simulink model "Measure_collection_Vf_W"  (R2021b)
settings: Solver=FixedStepAuto  StartTime=0.0  StopTime=200  FixedStep=1e-2  MaxStep=1e-1  RelTol=1e-2
values from neighbouring files (symbols this model uses):
  Ba = 0.02*ones(3,1)    [sensors_model.m]
  Bg = 5*ones(3,1)    [sensors_model.m]
undefined symbols (not defined in the file or in its folder): B, Spline
libraries: robotcorelib x10
settings Model: Creator=vince  LastModifiedBy=pierg

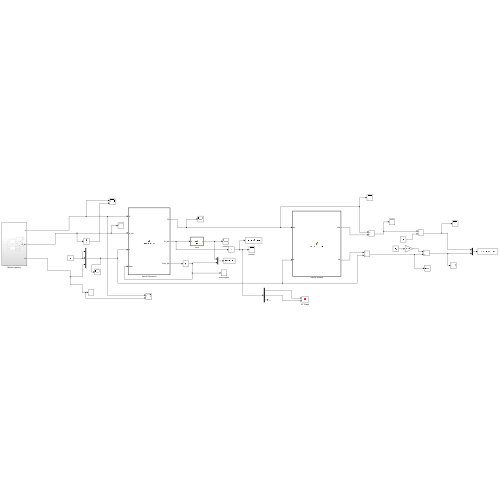
[thumbnail: Simulink's stored preview of the top-level diagram]
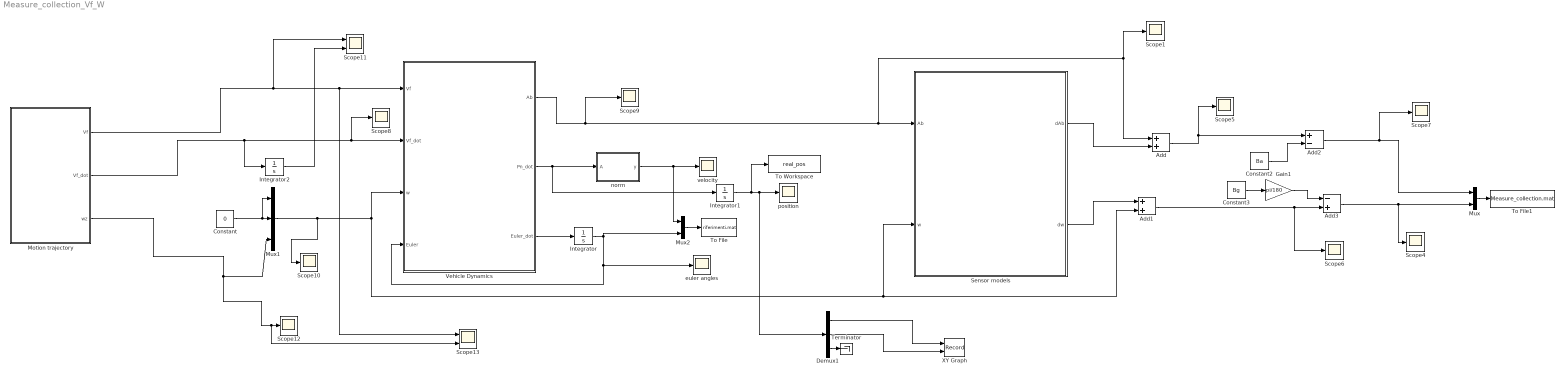
== system Measure_collection_Vf_W ==
  Add : Sum
  Add1 : Sum
  Add2 : Sum  Inputs=+-
  Add3 : Sum  Inputs=-+
  Constant : Constant  Value=0
  Constant2 : Constant  Value=Ba
  Constant3 : Constant  Value=Bg
  Demux1 : Demux  Outputs=3
  Gain1 : Gain  Gain=pi/180
  Integrator : Integrator  InitialCondition=[0 0 pi/2]'
  Integrator1 : Integrator  InitialCondition=[0 0 0]'
  Integrator2 : Integrator
  Motion trajectory : Subsystem
  Mux : Mux  Inputs=2
  Mux1 : Mux  Inputs=3
  Mux2 : Mux  Inputs=2
  Scope{1,4..10,12} (9 alike) : Scope
  Scope11 : Scope  NumInputPorts=2
  Scope13 : Scope  NumInputPorts=2
  Sensor models : MATLAB Function  TreatAsAtomicUnit=on
  Terminator : Terminator
  To File : ToFile  Filename=riferimenti.mat  MatrixName=ground_truth
  To File1 : ToFile  Filename=Measure_collection.mat  MatrixName=measure
  To Workspace : ToWorkspace  VariableName=real_pos  SaveFormat=Structure With Time  SampleTime=-1
  Vehicle Dynamics : MATLAB Function  TreatAsAtomicUnit=on
  XY Graph : Record  FileSettingsInternal="{\"entries\":[{\"content\":{\"excelSettings\":{\"content\":{},\"type\":\"Streamout.ExcelSettings\"}},\"type\":\"Streamout.FileSettingStorage\",\"uuid\":\"d67d7959-5b69-43ab-8784-a510eb5570ce\"}],\"packageUris\":[\"http://schema.mathworks.com/mf0/streamout_blocks/R2020a\"],\"version\":\"1.0\"}"  Layout=[1 1]  SignalsInternal="{\"entries\":[{\"content\":{\"signals\":[{\"content\":{\"blockPath\":[\"Measure_collection_Vf_W/XY Graph\"],\"channel\":[],\"dimensions\":[1,1],\"domain\":\"Measure_collection_Vf_W/XY Graph\",\"lineColor\":\"#a2142f\",\"plots\":[1],\"port\":1,\"sid\":[\"\"],\"signalID\":8310,\"signalName\":\"Demux1:1\"},\"type\":\"RecordBlkView.Signal\",\"uuid\":\"d98b29fb-951e-4e16-8393-070bce4ed298\"},{\"content\":{\"blockPath\":[\"Measure_collection_Vf_W/XY Graph\"],\"channel\":[],\"dimensions\":[1,1],\"domain\":\"Measure_collection_Vf_W/XY Graph\",\"lineColor\":\"#139fff\",\"plots\":[1],\"port\":2,\"sid\":[\"\"],\"signalID\":8314,\"signalName\":\"Demux1:2\"},\"type\":\"RecordBlkView.Signal\",\"uuid\":\"cd6d549f-a1b7-4e28-9178-ba3033d08120\"}]},\"type\":\"RecordBlkView.InputSignals\",\"uuid\":\"81421917-7cfd-46e5-9d72-67f20ea953c8\"}],\"packageUris\":[\"http://schema.mathworks.com/mf0/streamout_blocks/R2020a\"],\"version\":\"1.0\"}"  VisualizationBindings="{\"xyplotplugin\":{\"info\":[{\"series\":[{\"bindingParametersList\":[{\"parameter\":\"X-Axis\",\"signalID\":8310,\"signalName\":\"Demux1:1\"},{\"parameter\":\"Y-Axis\",\"signalID\":8314,\"signalName\":\"Demux1:2\"}],\"seriesID\":35238}],\"subplotID\":1}]}}"  CompatibilityTag=XY
  euler angles : Scope
  norm : MATLAB Function  TreatAsAtomicUnit=on
  position : Scope
  velocity : Scope
  wires:
  Sensor models/1(dAb) -> Add/2
  Mux1/1 -> Scope10/1, Vehicle Dynamics/3(w), Sensor models/2(w), Add1/2
  Sensor models/2(dw) -> Add1/1
  Add/1 -> Add2/1, Scope5/1
  Mux/1 -> To File1/1
  Vehicle Dynamics/3(Euler_dot) -> Integrator/1
  Vehicle Dynamics/2(Pn_dot) -> norm/1(A), Integrator1/1
  Integrator/1 -> Mux2/2, Vehicle Dynamics/4(Euler), euler angles/1
  Add1/1 -> Scope6/1, Add3/2
  Vehicle Dynamics/1(Ab) -> Scope9/1, Scope1/1, Add/1, Sensor models/1(Ab)
  Constant2/1 -> Add2/2
  Add2/1 -> Scope7/1, Mux/1
  Add3/1 -> Scope4/1, Mux/2
  Constant3/1 -> Gain1/1
  Gain1/1 -> Add3/1
  Motion trajectory/2(Vf_dot) -> Integrator2/1, Scope8/1, Vehicle Dynamics/2(Vf_dot)
  Constant/1 -> Mux1/1, Mux1/2
  Motion trajectory/3(wz) -> Mux1/3, Scope13/2, Scope12/1
  Motion trajectory/1(Vf) -> Scope11/1, Vehicle Dynamics/1(Vf), Scope13/1
  Integrator2/1 -> Scope11/2
  norm/1(y) -> Mux2/1, velocity/1
  Demux1/1 -> XY Graph/1
  Integrator1/1 -> To Workspace/1, Demux1/1, position/1
  Demux1/2 -> XY Graph/2
  Demux1/3 -> Terminator/1
  Mux2/1 -> To File/1

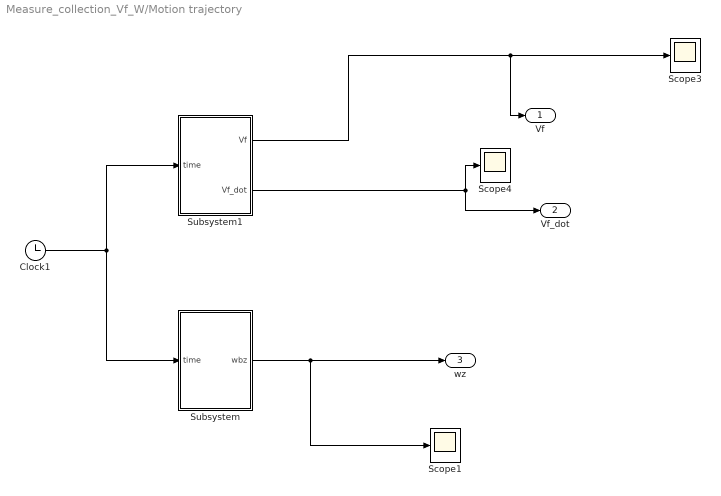
== system Measure_collection_Vf_W/Motion trajectory ==
  Clock1 : Clock
  Scope1 : Scope
  Scope3 : Scope
  Scope4 : Scope
  Subsystem : Subsystem
  Subsystem1 : Subsystem
  Vf : Outport
  Vf_dot : Outport  Port=2
  wz : Outport  Port=3
  wires:
  Clock1/1 -> Subsystem1/1(time), Subsystem/1(time)
  Subsystem1/2(Vf_dot) -> Scope4/1, Vf_dot/1
  Subsystem1/1(Vf) -> Vf/1, Scope3/1
  Subsystem/1(wbz) -> Scope1/1, wz/1

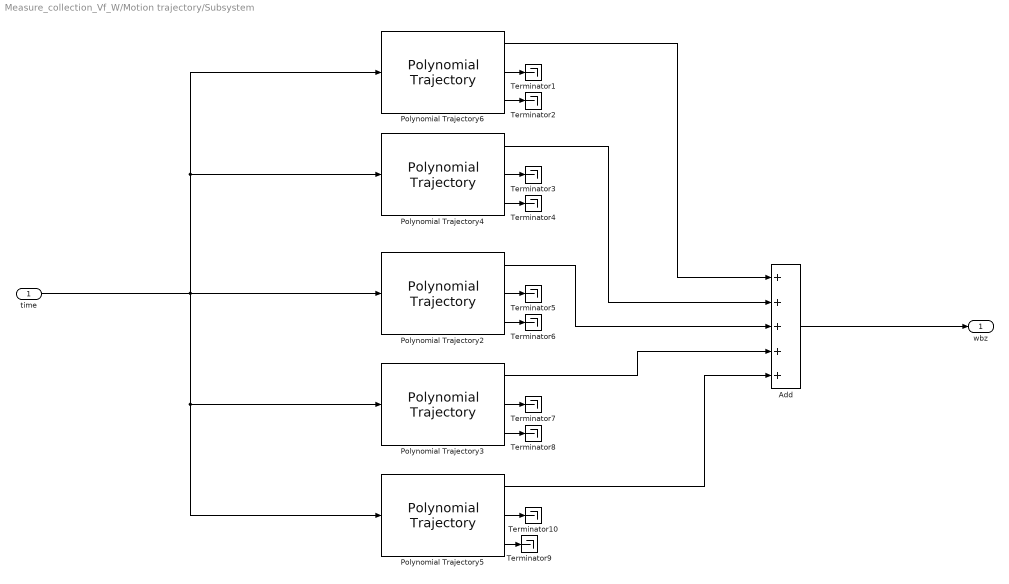
== system Measure_collection_Vf_W/Motion trajectory/Subsystem ==
  time : Inport
  Add : Sum  Inputs=+++++
  Polynomial Trajectory2 : robotcorelib/Polynomial Trajectory  WaypointSource=Internal  Waypoints=wz_des_3  TimePoints=[ 0, 2, 4, , ]  TimeInterval=[75, 115]  Method=B-Spline  ParameterSource=Internal  VelocityBoundaryCondition=zeros( 1, 5 )  AccelerationBoundaryCondition=zeros( 2, 5 )  SimulateUsing=Interpreted execution
  Polynomial Trajectory3 : robotcorelib/Polynomial Trajectory  WaypointSource=Internal  Waypoints=wz_des_4  TimePoints=[ 0, 2, 4, , ]  TimeInterval=[115, 155]  Method=B-Spline  ParameterSource=Internal  VelocityBoundaryCondition=zeros( 1, 5 )  AccelerationBoundaryCondition=zeros( 2, 5 )  SimulateUsing=Interpreted execution
  Polynomial Trajectory4 : robotcorelib/Polynomial Trajectory  WaypointSource=Internal  Waypoints=wz_des_2  TimePoints=[ 0, 2, 4, , ]  TimeInterval=[35, 75]  Method=B-Spline  ParameterSource=Internal  VelocityBoundaryCondition=zeros( 1, 5 )  AccelerationBoundaryCondition=zeros( 2, 5 )  SimulateUsing=Interpreted execution
  Polynomial Trajectory5 : robotcorelib/Polynomial Trajectory  WaypointSource=Internal  Waypoints=wz_des_5  TimePoints=[ 0, 2, 4, , ]  TimeInterval=[155, 200]  Method=B-Spline  ParameterSource=Internal  VelocityBoundaryCondition=zeros( 1, 5 )  AccelerationBoundaryCondition=zeros( 2, 5 )  SimulateUsing=Interpreted execution
  Polynomial Trajectory6 : robotcorelib/Polynomial Trajectory  WaypointSource=Internal  Waypoints=wz_des_1  TimePoints=[ 0, 2, 4, , ]  TimeInterval=[0, 35]  Method=B-Spline  ParameterSource=Internal  VelocityBoundaryCondition=zeros( 1, 5 )  AccelerationBoundaryCondition=zeros( 2, 5 )  SimulateUsing=Interpreted execution
  Terminator{1..10} (10 alike) : Terminator
  wbz : Outport
  wires:
  Polynomial Trajectory2/2 -> Terminator5/1
  Polynomial Trajectory6/1 -> Add/1
  Polynomial Trajectory3/1 -> Add/4
  Polynomial Trajectory4/1 -> Add/2
  Polynomial Trajectory3/3 -> Terminator8/1
  Polynomial Trajectory5/3 -> Terminator9/1
  Polynomial Trajectory6/3 -> Terminator2/1
  Polynomial Trajectory4/2 -> Terminator3/1
  Polynomial Trajectory2/1 -> Add/3
  Polynomial Trajectory5/1 -> Add/5
  Polynomial Trajectory3/2 -> Terminator7/1
  Polynomial Trajectory2/3 -> Terminator6/1
  Polynomial Trajectory5/2 -> Terminator10/1
  Polynomial Trajectory6/2 -> Terminator1/1
  Polynomial Trajectory4/3 -> Terminator4/1
  Add/1 -> wbz/1
  time/1 -> Polynomial Trajectory5/1, Polynomial Trajectory3/1, Polynomial Trajectory2/1, Polynomial Trajectory6/1, Polynomial Trajectory4/1

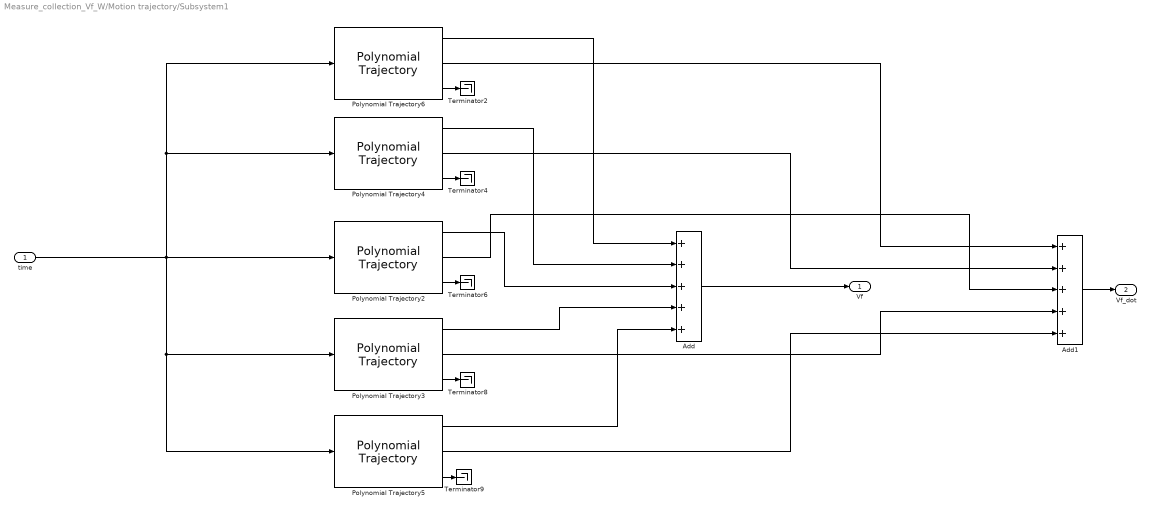
== system Measure_collection_Vf_W/Motion trajectory/Subsystem1 ==
  time : Inport
  Add : Sum  Inputs=+++++
  Add1 : Sum  Inputs=+++++
  Polynomial Trajectory2 : robotcorelib/Polynomial Trajectory  WaypointSource=Internal  Waypoints=Vf_des_3  TimePoints=[ 0, 2, 4, , ]  TimeInterval=[75, 115]  Method=B-Spline  ParameterSource=Internal  VelocityBoundaryCondition=zeros( 1, 5 )  AccelerationBoundaryCondition=zeros( 2, 5 )  SimulateUsing=Interpreted execution
  Polynomial Trajectory3 : robotcorelib/Polynomial Trajectory  WaypointSource=Internal  Waypoints=Vf_des_4  TimePoints=[ 0, 2, 4, , ]  TimeInterval=[115, 155]  Method=B-Spline  ParameterSource=Internal  VelocityBoundaryCondition=zeros( 1, 5 )  AccelerationBoundaryCondition=zeros( 2, 5 )  SimulateUsing=Interpreted execution
  Polynomial Trajectory4 : robotcorelib/Polynomial Trajectory  WaypointSource=Internal  Waypoints=Vf_des_2  TimePoints=[ 0, 2, 4, , ]  TimeInterval=[35, 75]  Method=B-Spline  ParameterSource=Internal  VelocityBoundaryCondition=zeros( 1, 5 )  AccelerationBoundaryCondition=zeros( 2, 5 )  SimulateUsing=Interpreted execution
  Polynomial Trajectory5 : robotcorelib/Polynomial Trajectory  WaypointSource=Internal  Waypoints=Vf_des_5  TimePoints=[ 0, 2, 4, , ]  TimeInterval=[155, 200]  Method=B-Spline  ParameterSource=Internal  VelocityBoundaryCondition=zeros( 1, 5 )  AccelerationBoundaryCondition=zeros( 2, 5 )  SimulateUsing=Interpreted execution
  Polynomial Trajectory6 : robotcorelib/Polynomial Trajectory  WaypointSource=Internal  Waypoints=Vf_des_1  TimePoints=[ 0, 2, 4, , ]  TimeInterval=[0, 35]  Method=B-Spline  ParameterSource=Internal  VelocityBoundaryCondition=zeros( 1, 5 )  AccelerationBoundaryCondition=zeros( 2, 5 )  SimulateUsing=Interpreted execution
  Terminator{2,4,6,8..9} (5 alike) : Terminator
  Vf : Outport
  Vf_dot : Outport  Port=2
  wires:
  Polynomial Trajectory2/2 -> Add1/3
  Polynomial Trajectory6/1 -> Add/1
  Polynomial Trajectory3/1 -> Add/4
  Polynomial Trajectory4/1 -> Add/2
  Polynomial Trajectory3/3 -> Terminator8/1
  Polynomial Trajectory5/3 -> Terminator9/1
  Polynomial Trajectory6/3 -> Terminator2/1
  Polynomial Trajectory4/2 -> Add1/2
  Polynomial Trajectory2/1 -> Add/3
  Polynomial Trajectory5/1 -> Add/5
  Polynomial Trajectory3/2 -> Add1/4
  Polynomial Trajectory2/3 -> Terminator6/1
  Polynomial Trajectory5/2 -> Add1/5
  Polynomial Trajectory6/2 -> Add1/1
  Polynomial Trajectory4/3 -> Terminator4/1
  Add/1 -> Vf/1
  time/1 -> Polynomial Trajectory5/1, Polynomial Trajectory3/1, Polynomial Trajectory2/1, Polynomial Trajectory6/1, Polynomial Trajectory4/1
  Add1/1 -> Vf_dot/1

== matlab function Measure_collection_Vf_W/Sensor models ==
  settings: updateMethod=DISCRETE
  data: Ab input; dAb output; w input; dw output
function [dAb, dw] = sensors_model(Ab, w)

%% Parameters

% Accelerometer
Ba = 0.02; % m/s^2
SFa = 0.05;
MISa = 0.1; % deg
stdv_a = 4*0.0055; % standard deviation
Wna = stdv_a*randn(3,1); % White Noise

Sa = [SFa MISa MISa;
      MISa SFa MISa;
      MISa MISa SFa];

% Compensazione gravità
g = 9.81;
Ab_g = Ab + [0 0 g]';

% Gyros
Bg = 5*pi/180; % deg/s
SFg = 0;
MISg = 0.1*pi/180; % deg
stdv_g = 0.6325*pi/180; % standard deviation
Wng = stdv_g*randn(3,1); % White Noise

Sg = [SFg MISg MISg;
      MISg SFg MISg;
      MISg MISg SFg];

%% Models

% Accelerometer
dAb = Ba*ones(3,1) + Sa * Ab_g + Wna;

% Gyros
dw = Bg*ones(3,1) + Sg * w + Wng;

== matlab function Measure_collection_Vf_W/Vehicle Dynamics ==
  data: Vf input; Vf_dot input; w input; Euler input; Ab output; Pn_dot output; Euler_dot output
function [Ab, Pn_dot, Euler_dot] = Vehicle_model(Vf, Vf_dot, w, Euler)
%% Land Vehicle Dynamic model
% x_dot is the derivative of x
wbx = w(1);
wby = w(2);
wbz = w(3);

% Euler angles
phi = Euler(1);
theta = Euler(2);
psi = Euler(3);

% Constant
g = 9.81;

% Model
Abx = Vf_dot + g*sin(theta);
Aby = Vf*wbz - g*sin(phi)*cos(theta);
Abz = -Vf*wby - g*cos(phi)*cos(theta);
phi_dot = wbx + sin(phi)*tan(theta)*wby + cos(phi)*tan(theta)*wbz;
theta_dot = cos(phi)*wby - sin(phi)*wbz;
psi_dot = sin(phi)/cos(theta)*wby + cos(phi)/cos(theta) * wbz;
Pnn_dot = Vf*cos(theta)*cos(psi);
Pne_dot = Vf*cos(theta)*sin(psi);
Pnd_dot = Vf*sin(theta);

Ab = [Abx, Aby, Abz]';
Euler_dot = [phi_dot, theta_dot, psi_dot]';
Pn_dot = [Pnn_dot, Pne_dot, Pnd_dot]';

== matlab function Measure_collection_Vf_W/norm ==
  data: A input; y output
function y = fcn(A)
y = norm(A);
